simulink model "angular_velocity_controller"  (R2019b)
settings: Solver=VariableStepAuto  StartTime=0.0  StopTime=10.0  RelTol=1e-3
values from neighbouring files (symbols this model uses):
  d1 = 2    [PlotScript.m]
  p1 = 4    [PlotScript.m]
undefined symbols (not defined in the file or in its folder): DiscIntNeverNeededParam
libraries: simulink x1
settings Model: Creator=alilf  LastModifiedBy=alilf

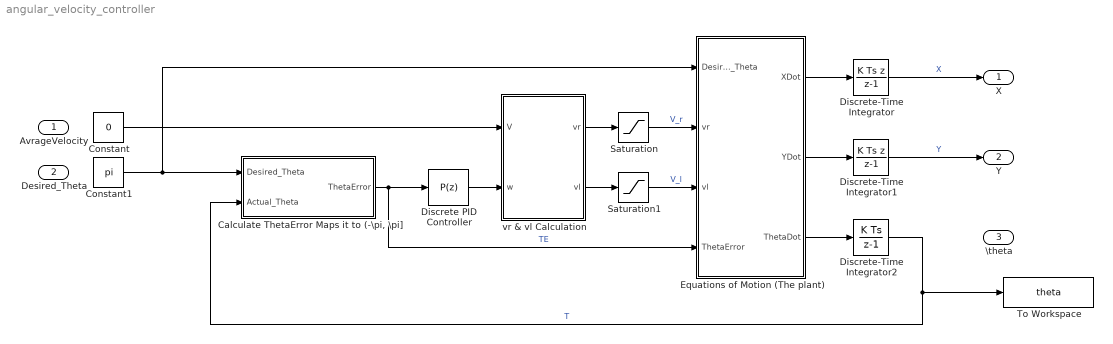
== system angular_velocity_controller ==
  AvrageVelocity : Inport
  Desired_Theta : Inport  Port=2
  "Calculate ThetaError Maps it to (-\\pi, \\pi]" : MATLAB Function  TreatAsAtomicUnit=on
  Constant : Constant  Value=0  SampleTime=0.1
  Constant1 : Constant  Value=pi  SampleTime=0.1
  Discrete PID Controller : simulink/Continuous/PID Controller  Controller=P  Form=Parallel  TimeDomain=Discrete-time  SampleTime=0.1  IntegratorMethod=Forward Euler  FilterMethod=Forward Euler  ControllerParametersSource=internal  P=p1  I=1  D=d1  UseFilter=on  N=100  TunerSelectOption=Transfer Function Based (PID Tuner App)  InitialConditionSource=internal  InitialConditionForIntegrator=0  InitialConditionForFilter=0  DifferentiatorICPrevScaledInput=0  ExternalReset=none  TrackingMode=off  Kt=1  LimitOutput=off  UpperSaturationLimit=inf  LowerSaturationLimit=-inf  LinearizeAsGain=off  AntiWindupMode=none  Kb=1  POutMin=[]  POutMax=[]  IOutMin=[]  IOutMax=[]  DOutMin=[]  DOutMax=[]  NOutMin=[]  NOutMax=[]  SumOutMin=[]  SumOutMax=[]  SaturationOutMin=[]  SaturationOutMax=[]  PParamMin=[]  PParamMax=[]  IParamMin=[]  IParamMax=[]  DParamMin=[]  DParamMax=[]  NParamMin=[]  NParamMax=[]  KbParamMin=[]  KbParamMax=[]  KtParamMin=[]  KtParamMax=[]  KbOutMin=[]  KbOutMax=[]  KtOutMin=[]  KtOutMax=[]  IntegratorOutMin=[]  IntegratorOutMax=[]  FilterOutMin=[]  FilterOutMax=[]  SumI1OutMin=[]  SumI1OutMax=[]  SumI2OutMin=[]  SumI2OutMax=[]  SumI3OutMin=[]  SumI3OutMax=[]  SumI4OutMin=[]  SumI4OutMax=[]  SumDOutMin=[]  SumDOutMax=[]  DifferentiatorOutMin=[]  DifferentiatorOutMax=[]  FilterDiffOutCoefMin=[]  FilterDiffOutCoefMax=[]  ReciprocalOutMin=[]  ReciprocalOutMax=[]  SumDenOutMin=[]  SumDenOutMax=[]  SumNumOutMin=[]  SumNumOutMax=[]  DivideOutMin=[]  DivideOutMax=[]  IntegratorContinuousStateAttributes=''  IntegratorStateMustResolveToSignalObject=off  IntegratorRTWStateStorageClass=Auto  FilterContinuousStateAttributes=''  FilterStateMustResolveToSignalObject=off  FilterRTWStateStorageClass=Auto  ParallelPVariant=InternalParameters  IdealPVariant=Disabled  IVariant=Disabled  DVariant=Disabled  IntegratorVariant=Disabled  SatVariant=Disabled  AWVariant=Disabled  PCopyVariant=Disabled  TRVariant=Disabled  FdbkBlocksVariant=Forward  IdealPFdbkVariant=Disabled  SatFdbkVariant=Disabled  DerivativeFilterVariant=Disabled  NVariant=Disabled  NCopyVariant=Disabled_SignalSpec  FilterICVariant=Disabled  IntegratorICVariant=Disabled  ExternalResetVariant=Disabled  TRSumVariant=Passthrough  SumFdbkVariant=Disabled  SumVariant=Passthrough_P
  "Discrete-Time Integrator " : DiscreteIntegrator  IntegratorMethod=Integration: Backward Euler  SampleTime=0.1  ICPrevOutput=DiscIntNeverNeededParam  ICPrevScaledInput=DiscIntNeverNeededParam
  "Discrete-Time Integrator1 " : DiscreteIntegrator  IntegratorMethod=Integration: Backward Euler  SampleTime=0.1  ICPrevOutput=DiscIntNeverNeededParam  ICPrevScaledInput=DiscIntNeverNeededParam
  "Discrete-Time Integrator2 " : DiscreteIntegrator  SampleTime=0.1  ICPrevOutput=DiscIntNeverNeededParam  ICPrevScaledInput=DiscIntNeverNeededParam
  Equations of Motion (The plant) : MATLAB Function  TreatAsAtomicUnit=on  SystemSampleTime=0.1
  "Saturation " : Saturate  UpperLimit=10  LowerLimit=-10
  "Saturation1 " : Saturate  UpperLimit=10  LowerLimit=-10
  To Workspace : ToWorkspace  VariableName=theta  SaveFormat=Timeseries  SampleTime=-1
  vr & vl Calculation : MATLAB Function  TreatAsAtomicUnit=on  SystemSampleTime=0.1
  X : Outport
  Y : Outport  Port=2
  \theta : Outport  Port=3
  wires:
  Equations of Motion (The plant)/2(YDot) -> "Discrete-Time Integrator1 "/1
  "Discrete-Time Integrator1 "/1 -> Y/1  "Y"
  "Saturation "/1 -> Equations of Motion (The plant)/2(vr)  "V_r"
  Discrete PID Controller/1 -> vr & vl Calculation/2(w)
  "Discrete-Time Integrator2 "/1 -> To Workspace/1, "Calculate ThetaError Maps it to (-\\pi, \\pi]"/2(Actual_Theta)  "T"
  Equations of Motion (The plant)/1(XDot) -> "Discrete-Time Integrator "/1
  vr & vl Calculation/1(vr) -> "Saturation "/1
  "Calculate ThetaError Maps it to (-\\pi, \\pi]"/1(ThetaError) -> Equations of Motion (The plant)/4(ThetaError), Discrete PID Controller/1  "TE"
  vr & vl Calculation/2(vl) -> "Saturation1 "/1
  "Saturation1 "/1 -> Equations of Motion (The plant)/3(vl)  "V_l"
  "Discrete-Time Integrator "/1 -> X/1  "X"
  Equations of Motion (The plant)/3(ThetaDot) -> "Discrete-Time Integrator2 "/1
  Constant/1 -> vr & vl Calculation/1(V)
  Constant1/1 -> Equations of Motion (The plant)/1(Desired_Theta), "Calculate ThetaError Maps it to (-\\pi, \\pi]"/1(Desired_Theta)

== matlab function angular_velocity_controller/Equations of Motion (The plant) ==
  data: Desired_Theta input; vr input; XDot output; vl input; YDot output; ThetaDot output; ThetaError input
function [XDot, YDot, ThetaDot] = fcn(Desired_Theta, vr, vl, ThetaError )
L = 21; %the width of the robot in [cm]
Theta = Desired_Theta - ThetaError;
V = vr + vl;
XDot = V * cos(Theta) / 2;
YDot = V * sin(Theta) / 2;
ThetaDot = (vr - vl) / L;

== matlab function angular_velocity_controller/vr & vl Calculation ==
  data: V input; vr output; w input; vl output
function [vr, vl] = fcn(V,w)
L = 21; %the width of the robot in [cm]
vr = V + L*w/2;
vl = V - L*w/2;

== matlab function angular_velocity_controller/Calculate ThetaError Maps it to (-\pi, \pi] ==
  data: Desired_Theta input; ThetaError output; Actual_Theta input
function ThetaError = fcn(Desired_Theta, Actual_Theta)
%Calculate ThetaError
%Maps it to (-\pi, \pi]

TDiff = (Desired_Theta - Actual_Theta);
ThetaError = atan2(sin(TDiff), cos(TDiff));
